simulink model "integral_01"  (R2021b)
settings: Solver=VariableStepAuto  StartTime=0.0  StopTime=1  RelTol=1e-3
settings Model: Creator=86195  LastModifiedBy=86195

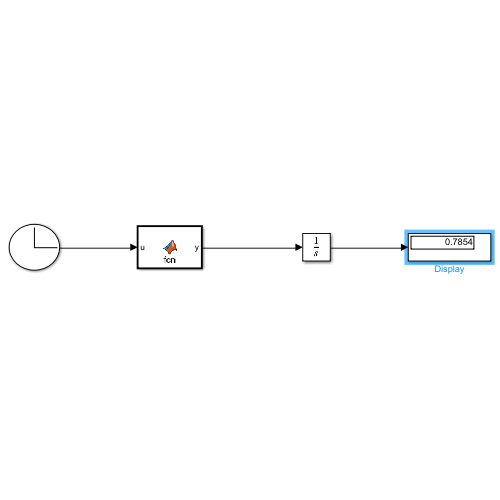
[thumbnail: Simulink's stored preview of the top-level diagram]
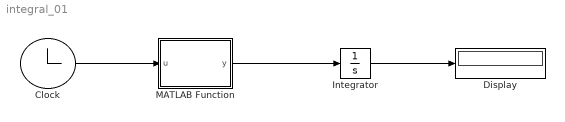
== system integral_01 ==
  Clock : Clock
  Display : Display
  Integrator : Integrator
  MATLAB Function : MATLAB Function  TreatAsAtomicUnit=on
  wires:
  Clock/1 -> MATLAB Function/1(u)
  MATLAB Function/1(y) -> Integrator/1
  Integrator/1 -> Display/1

== matlab function integral_01/MATLAB Function ==
  data: u input; y output
function y = fcn(u)

y = sqrt(1-u*u);
